simulink model "controller"  (Simulink 9.0)
settings: Solver=FixedStepDiscrete  StartTime=0.0  StopTime=CONFIG.TEnd  FixedStep=CONFIG.TS  RelTol=1e-3  EnableMultiTasking=on
InitFcn:
  | clc
  | cd(fileparts(which(bdroot)));
  | initTrqBalancingSeeSaw;
values from neighbouring files (symbols this model uses):
  LEFT_RIGHT_FOOT_IN_CONTACT = [1;1]    [initTrqBalancingSeeSaw.m]
undefined symbols (not defined in the file or in its folder): bVectorConstraints, Config, CONFIG, ConstraintsMatrix, directionOfOscillation, gain, noOscillationTime, referenceParams, reg, ROBOT_DOF, sat, seesaw
undefined symbols (not defined in the file): FRAMES
libraries: WBToolboxLibrary x47
(part 2 of 2)

== matlab function Robot and seesaw state/Seesaw orientation and angVelocity/Seesaw orientation and ang velocity from IMU seesaw/Seesaw rotation with IMU_seesaw/Correct IMU orientation ==
  data: wImu_data input double; w_data output double; seesaw parameter double
function w_data = rotateImuWorldFrameFCN(wImu_data,seesaw)

w_data = rotateImuWorldFrame(wImu_data,seesaw);

end

== matlab function Robot and seesaw state/Seesaw orientation and angVelocity/Seesaw orientation and ang velocity from IMU seesaw/Seesaw rotation with IMU_seesaw/theta_x from acc ==
  data: acc input double; theta_x output double
function theta_x = arctangent(acc)

% theta_x (seesaw roll) in radians
theta_x = atan2(acc(2),acc(3));

end

== matlab function Robot and seesaw state/Seesaw orientation and angVelocity/Seesaw orientation and ang velocity from IMU seesaw/Seesaw rotation with IMU_seesaw/Rotation matrix from angles ==
  data: angles input double; w_R_s output double
function w_R_s = rotationMatrixFromAngles(angles)

% See http://wiki.icub.org/images/8/82/XsensMtx.pdf page 12
w_R_s = rotz(angles(3))*roty(angles(2))*rotx(angles(1));

end

== matlab function Robot and seesaw state/Compute base velocity/evaluateBaseVelocity ==
  data: v_base output double; J_fixedLink input double; w_R_s input double; dqj input double; s_omega input double; seesaw parameter double; reg parameter double
function v_base  = computeBaseVelocityFCN(J_fixedLink,w_R_s,dqj,s_omega,seesaw,reg)

    v_base = computeBaseVelocitySeesaw(J_fixedLink,w_R_s,dqj,s_omega,seesaw,reg);

end

== matlab function Robot and seesaw state/Compute w_H_b  /Compute w_H_fixedLink/fixedLink w.r.t the world frame ==
  data: w_R_s input double; w_H_fixedLink output double; seesaw parameter double
function w_H_fixedLink = computeTransFromFixedLinkToWorldFCN(w_R_s,seesaw)

w_H_fixedLink = computeTransFromFixedLinkToWorld(w_R_s,seesaw);

end

== matlab function Balancing controller and QP solver/  integral of H_r /MATLAB Function ==
  data: qjErr input double; JL input double; JR input double; vbEquivalent output double; reg parameter double; activeFeetConstraints input double
function vbEquivalent = generateReferencesForH(qjErr,JL,JR,reg,activeFeetConstraints)

% The approximation of integral of angular momentum is given by:
%
%    H_approx = JG(qRef)*(qj-qjDes)
%
% It is assumed here that one of the feet is always on ground at time t=0
% 
if activeFeetConstraints(1) == 1
    
    pinvJb             = (transpose(JL(:,1:6))*JL(:,1:6) + reg.pinvTolVb*eye(6))\transpose(JL(:,1:6));
    vbEquivalent       = -pinvJb*JL(:,7:end)*qjErr;
else
    
    pinvJb             = (transpose(JR(:,1:6))*JR(:,1:6) + reg.pinvTolVb*eye(6))\transpose(JR(:,1:6));
    vbEquivalent       = -pinvJb*JR(:,7:end)*qjErr;
end
end
